simulink model "FM_modelasion"  (R2016b)
settings: Solver=VariableStepAuto  StartTime=0.0  StopTime=inf  FixedStep=.0002  MaxStep=0.00005  RelTol=1e-4  EnableMultiTasking=on
libraries: simulink_extras x3, dsparch4 x2, dspsrcs4 x2, commsynccomp2 x2
settings Model: Creator=Asus  LastModifiedBy=Asus
settings DataIOCC: LimitDataPoints=on  SaveOutput=off  SaveTime=off
settings OptimizationCC: ExpressionDepthLimit=2147483647  LifeSpan=1
settings DebuggingCC: UnderspecifiedInitializationDetection=Classic  MergeDetectMultiDrivingBlocksExec=none  FcnCallInpInsideContextMsg=warning  AllowSymbolicDim=off  StateNameClashWarn=warning  SFUnexpectedBacktrackingDiag=warning  SFNoUnconditionalDefaultTransitionDiag=warning  SFExecutionAtInitializationDiag=none
settings GRTTargetCC: TargetLangStandard=C89/C90 (ANSI)  GeneratePreprocessorConditionals=Disable all  CombineOutputUpdateFcns=off  GRTInterface=on

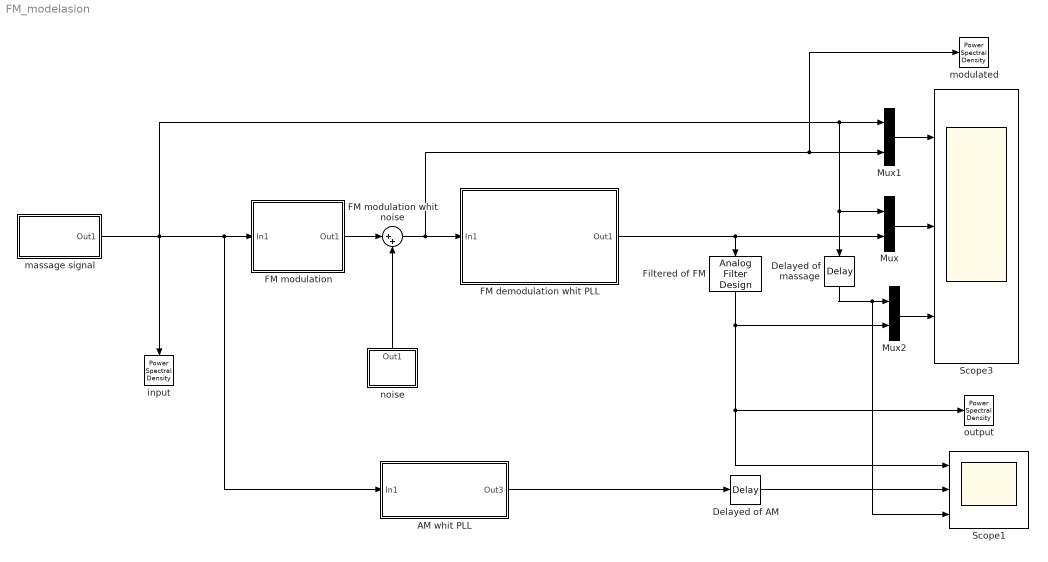
== system FM_modelasion ==
  " Filtered of FM" : dsparch4/Analog Filter Design  method=Butterworth  filttype=Lowpass  N=8  Wlo=30*2*pi  Whi=80  Rp=2  Rs=40
  AM whit PLL : Subsystem
  Delayed of massage : TransportDelay  DelayTime=(2*pi/10)/22
  "Delayed of AM " : TransportDelay  DelayTime=(2*pi/10)/22
  FM demodulation whit PLL : Subsystem
  FM modulation : Subsystem
  FM modulation whit noise : Sum  Inputs=|++
  Mux : Mux  Inputs=2
  Mux1 : Mux  Inputs=2
  Mux2 : Mux  Inputs=2
  Scope1 : Scope  NumInputPorts=3
  Scope3 : Scope  NumInputPorts=3
  input : simulink_extras/Additional Sinks/Power Spectral Density  npts=128  fftpts=512  HowOften=64  sampleT=1/45
  "massage signal " : Subsystem
  modulated : simulink_extras/Additional Sinks/Power Spectral Density  npts=128  fftpts=512  HowOften=64  sampleT=1/5000
  noise : Subsystem
  output : simulink_extras/Additional Sinks/Power Spectral Density  npts=128  fftpts=512  HowOften=64  sampleT=1/45
  wires:
  "massage signal "/1(Out1) -> input/1, Delayed of massage/1, Mux/1, Mux1/1, AM whit PLL/1(In1), FM modulation/1(In1)
  Mux/1 -> Scope3/2
  Mux1/1 -> Scope3/1
  FM demodulation whit PLL/1(Out1) -> Mux/2, " Filtered of FM"/1
  Mux2/1 -> Scope3/3
  FM modulation/1(Out1) -> FM modulation whit noise/1
  FM modulation whit noise/1 -> FM demodulation whit PLL/1(In1), modulated/1, Mux1/2
  Delayed of massage/1 -> Scope1/3, Mux2/1
  " Filtered of FM"/1 -> output/1, Scope1/1, Mux2/2
  AM whit PLL/1(Out3) -> "Delayed of AM "/1
  "Delayed of AM "/1 -> Scope1/2
  noise/1(Out1) -> FM modulation whit noise/2

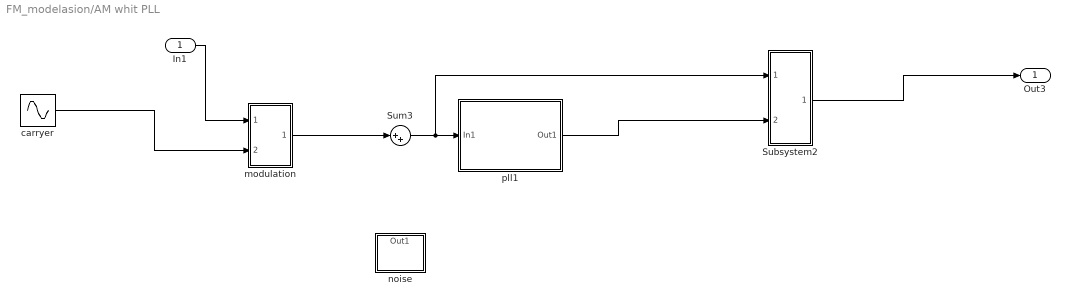
== system FM_modelasion/AM whit PLL ==
  In1 : Inport
  Subsystem2 : Subsystem
  Sum3 : Sum  Inputs=|++
  carryer : Sin  Frequency=1000*2*pi  SampleTime=0
  modulation : Subsystem
  noise : Subsystem
  pll1 : Subsystem
  Out3 : Outport
  wires:
  carryer/1 -> modulation/2(In2)
  Subsystem2/1(Out2) -> Out3/1
  pll1/1(Out1) -> Subsystem2/2(In2)
  Sum3/1 -> pll1/1(In1), Subsystem2/1(In1)
  modulation/1(Out1) -> Sum3/1
  In1/1 -> modulation/1(In1)

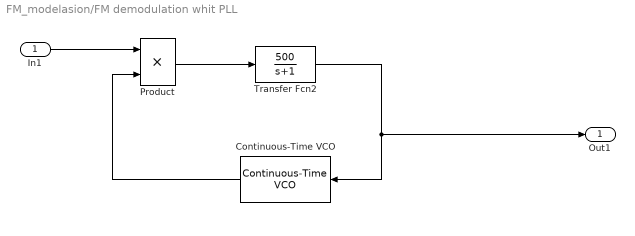
== system FM_modelasion/FM demodulation whit PLL ==
  In1 : Inport
  Continuous-Time VCO : commsynccomp2/Continuous-Time VCO  Ac=1  Fc=1000  Kc=200  Ph=0
  Product : Product
  Transfer Fcn2 : TransferFcn  Numerator=[500]  Denominator=[1 1]
  Out1 : Outport
  wires:
  In1/1 -> Product/1
  Continuous-Time VCO/1 -> Product/2
  Product/1 -> Transfer Fcn2/1
  Transfer Fcn2/1 -> Out1/1, Continuous-Time VCO/1

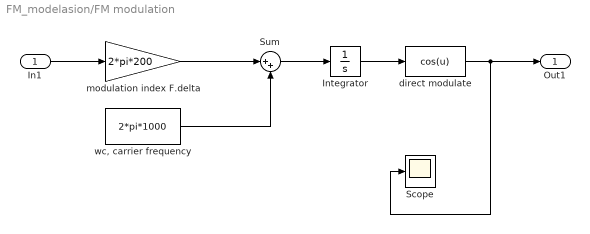
== system FM_modelasion/FM modulation ==
  In1 : Inport
  Integrator : Integrator  IgnoreLimit=on
  Scope : Scope
  Sum : Sum  Inputs=|++
  direct modulate : Fcn  Expr=cos(u)
  modulation index F.delta : Gain  Gain=2*pi*200
  "wc, carrier frequency" : Constant  Value=2*pi*1000
  Out1 : Outport
  wires:
  modulation index F.delta/1 -> Sum/1
  "wc, carrier frequency"/1 -> Sum/2
  Sum/1 -> Integrator/1
  Integrator/1 -> direct modulate/1
  direct modulate/1 -> Scope/1, Out1/1
  In1/1 -> modulation index F.delta/1

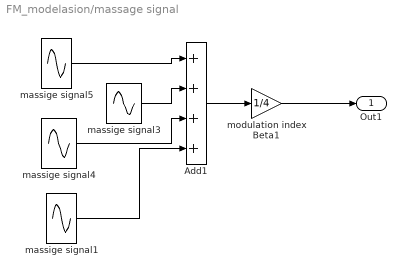
== system FM_modelasion/massage signal  ==
  Add1 : Sum  Inputs=++++
  massige signal1 : Sin  Frequency=11.33*2*pi  SampleTime=0
  massige signal3 : Sin  Frequency=13.333*2*pi  SampleTime=0
  massige signal4 : Sin  Frequency=10.54*2*pi  SampleTime=0
  massige signal5 : Sin  Frequency=8.37*2*pi  SampleTime=0
  modulation index Beta1 : Gain  Gain=1/4
  Out1 : Outport
  wires:
  modulation index Beta1/1 -> Out1/1
  Add1/1 -> modulation index Beta1/1
  massige signal4/1 -> Add1/3
  massige signal3/1 -> Add1/2
  massige signal5/1 -> Add1/1
  massige signal1/1 -> Add1/4

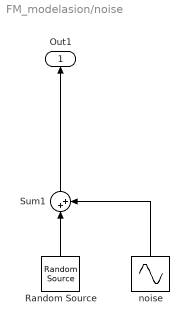
== system FM_modelasion/noise ==
  Random Source : dspsrcs4/Random Source  SrcType=Uniform  NormMethod=Ziggurat  CltLength=12  MinVal=-0.1  MaxVal=.1  MeanVal=0  VarVal=1  RepMode=Not repeatable  rawSeed=1  IsInherit=off  SampMode=Discrete  SampTime=0.0001  SampFrame=1  DataType=Double  OutComplex=Real  OutputFrames=off
  Sum1 : Sum  Inputs=|++
  noise : Sin  Amplitude=.1  Frequency=500.2*2*pi  SampleTime=0
  Out1 : Outport
  wires:
  Random Source/1 -> Sum1/1
  Sum1/1 -> Out1/1
  noise/1 -> Sum1/2

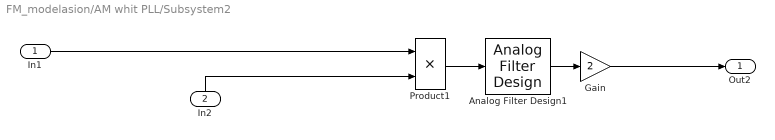
== system FM_modelasion/AM whit PLL/Subsystem2 ==
  In1 : Inport
  In2 : Inport  Port=2
  Analog Filter Design1 : dsparch4/Analog Filter Design  method=Elliptic  filttype=Lowpass  N=4  Wlo=15*2*pi  Whi=80  Rp=2  Rs=40
  Gain : Gain  Gain=2
  Product1 : Product
  Out2 : Outport
  wires:
  Analog Filter Design1/1 -> Gain/1
  Product1/1 -> Analog Filter Design1/1
  In2/1 -> Product1/2
  In1/1 -> Product1/1
  Gain/1 -> Out2/1

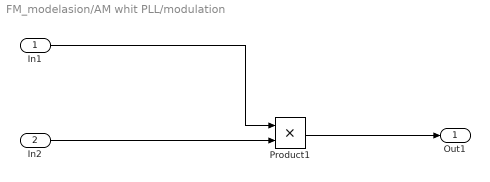
== system FM_modelasion/AM whit PLL/modulation ==
  In1 : Inport
  In2 : Inport  Port=2
  Product1 : Product
  Out1 : Outport
  wires:
  In2/1 -> Product1/2
  Product1/1 -> Out1/1
  In1/1 -> Product1/1

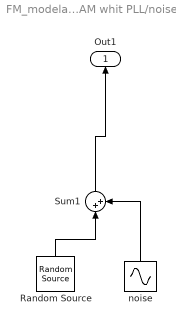
== system FM_modelasion/AM whit PLL/noise ==
  Random Source : dspsrcs4/Random Source  SrcType=Uniform  NormMethod=Ziggurat  CltLength=12  MinVal=-0.05  MaxVal=.05  MeanVal=0  VarVal=1  RepMode=Not repeatable  rawSeed=1  IsInherit=off  SampMode=Discrete  SampTime=0.0001  SampFrame=1  DataType=Double  OutComplex=Real  OutputFrames=off
  Sum1 : Sum  Inputs=|++
  noise : Sin  Amplitude=.05  Frequency=500.2*2*pi  SampleTime=0
  Out1 : Outport
  wires:
  Random Source/1 -> Sum1/1
  Sum1/1 -> Out1/1
  noise/1 -> Sum1/2

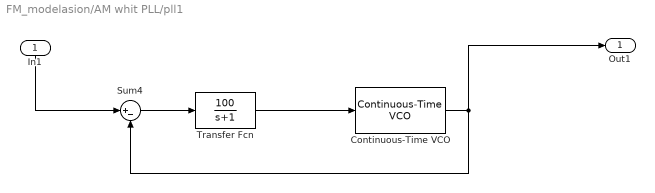
== system FM_modelasion/AM whit PLL/pll1 ==
  In1 : Inport
  Continuous-Time VCO : commsynccomp2/Continuous-Time VCO  Ac=1  Fc=1000  Kc=500  Ph=pi/2
  Sum4 : Sum  Inputs=|+-
  Transfer Fcn : TransferFcn  Numerator=[100]  Denominator=[1 1]
  Out1 : Outport
  wires:
  Continuous-Time VCO/1 -> Sum4/2, Out1/1
  Sum4/1 -> Transfer Fcn/1
  Transfer Fcn/1 -> Continuous-Time VCO/1
  In1/1 -> Sum4/1
